simulink model "ToLinDeltaTheta"  (R2019a)
settings: Solver=VariableStepAuto  StartTime=0.0  StopTime=10.0  RelTol=1e-3
values from neighbouring files (symbols this model uses):
  dPHRTrim = trimVal(1)    [mainProjetCADV_2a.m]
  dthrIdle = 0.1    [mainProjetCADV_2a.m]
  idelevator = 3    [mainProjetCADV_2a.m]
  thetaTrim = trimVal(3)    [mainProjetCADV_2a.m]
  uTrim = zeros(TOTAL_CMD, 1)    [mainProjetCADV_2a.m]
  xTrim = zeros(TOTAL_SV, 1)    [mainProjetCADV_2a.m]
undefined symbols (not defined in the file or in its folder): aircraftChosen, Kd, Ki, km, Kp, ms
settings Model: Creator=palotaba  LastModifiedBy=ulyss

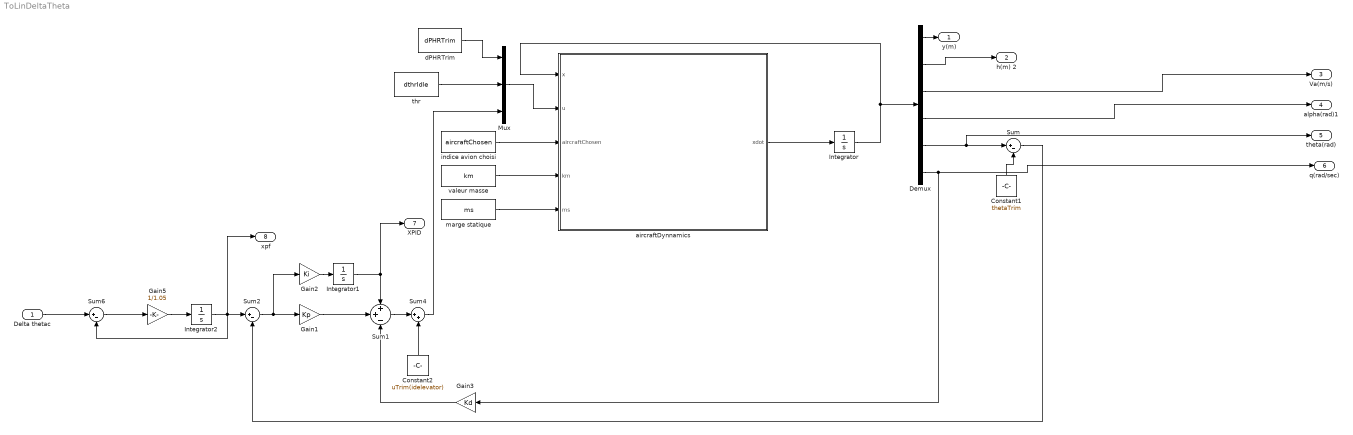
== system ToLinDeltaTheta ==
  "Delta thetac " : Inport
  Constant1 : Constant  Value=thetaTrim
  Constant2 : Constant  Value=uTrim(idelevator)
  Demux : Demux  Outputs=6
  Gain1 : Gain  Gain=Kp
  Gain2 : Gain  Gain=Ki
  Gain3 : Gain  Gain=Kd
  Gain5 : Gain  Gain=1/1.05
  Integrator : Integrator  InitialCondition=xTrim
  Integrator1 : Integrator
  Integrator2 : Integrator
  Mux : Mux  Inputs=3
  Sum : Sum  Inputs=|+-
  Sum1 : Sum  Inputs=++-
  Sum2 : Sum  Inputs=|+-
  Sum4 : Sum  Inputs=|++
  Sum6 : Sum  Inputs=|+-
  aircraftDynnamics : MATLAB Function  TreatAsAtomicUnit=on
  dPHRTrim : Constant  Value=dPHRTrim
  indice avion choisi : Constant  Value=aircraftChosen
  marge statique : Constant  Value=ms
  thr : Constant  Value=dthrIdle
  valeur masse : Constant  Value=km
  y(m) : Outport
  "h(m) 2 " : Outport  Port=2
  Va(m/s) : Outport  Port=3
  alpha(rad)1 : Outport  Port=4
  theta(rad) : Outport  Port=5
  q(rad/sec) : Outport  Port=6
  "XPID " : Outport  Port=7
  "xpf " : Outport  Port=8
  wires:
  marge statique/1 -> aircraftDynnamics/5(ms)
  Sum2/1 -> Gain2/1, Gain1/1
  Constant2/1 -> Sum4/2
  Demux/2 -> "h(m) 2 "/1
  Sum/1 -> Sum2/2
  thr/1 -> Mux/2
  Gain1/1 -> Sum1/2
  Sum1/1 -> Sum4/1
  Sum4/1 -> Mux/3
  Gain2/1 -> Integrator1/1
  indice avion choisi/1 -> aircraftDynnamics/3(aircraftChosen)
  Gain3/1 -> Sum1/3
  Demux/1 -> y(m)/1
  aircraftDynnamics/1(xdot) -> Integrator/1
  Integrator/1 -> aircraftDynnamics/1(x), Demux/1
  Integrator2/1 -> "xpf "/1, Sum6/2, Sum2/1
  Mux/1 -> aircraftDynnamics/2(u)
  dPHRTrim/1 -> Mux/1
  valeur masse/1 -> aircraftDynnamics/4(km)
  Constant1/1 -> Sum/2
  Integrator1/1 -> "XPID "/1, Sum1/1
  Demux/5 -> theta(rad)/1, Sum/1
  Demux/6 -> q(rad/sec)/1, Gain3/1
  Demux/3 -> Va(m/s)/1
  Demux/4 -> alpha(rad)1/1
  Gain5/1 -> Integrator2/1
  Sum6/1 -> Gain5/1
  "Delta thetac "/1 -> Sum6/1

== matlab function ToLinDeltaTheta/aircraftDynnamics ==
  data: x input; u input; xdot output; aircraftChosen input; km input; ms input
function xdot = aircraftDynamics(x,u, aircraftChosen,km,ms)
    TOTAL_SV = 6;
    xIn = zeros(TOTAL_SV,1);
    xIn = x;
    
	TOTAL_CMD = 3;
    uIn = zeros(TOTAL_CMD,1);
    uIn = u;
    
    xdot = utAcDynamicsFunction(xIn,uIn, aircraftChosen,km,ms);
end %aircraftDynamics
